simulink model "ECE545HW5_2"  (R2016a)
settings: Solver=VariableStepAuto  StartTime=0.0  StopTime=10.0  RelTol=1e-3
settings Model: Creator=clarke6  LastModifiedBy=clarke6

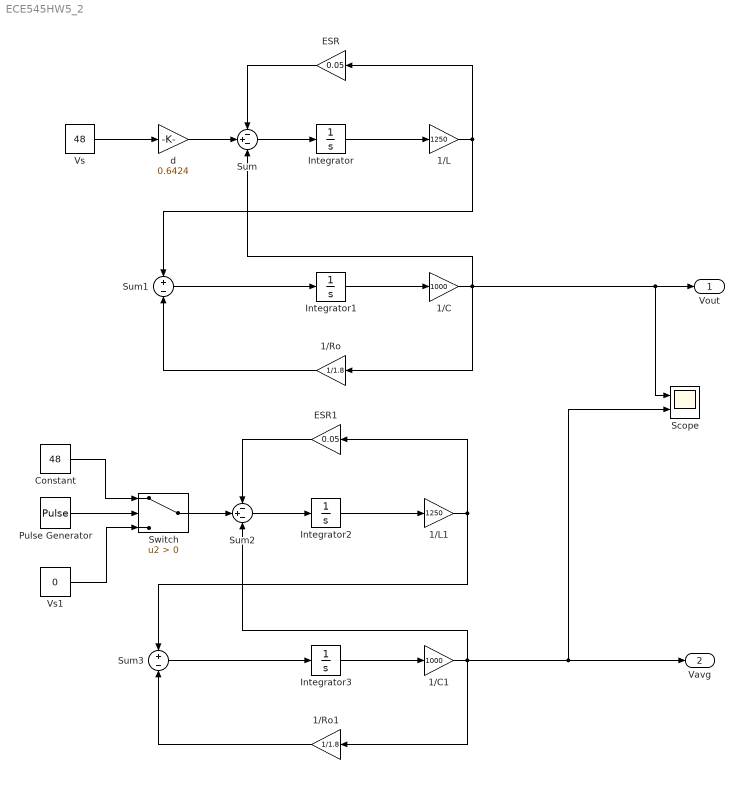
== system ECE545HW5_2 ==
  1/C : Gain  Gain=1000
  1/C1 : Gain  Gain=1000
  1/L : Gain  Gain=1250
  1/L1 : Gain  Gain=1250
  1/Ro : Gain  Gain=1/1.8
  1/Ro1 : Gain  Gain=1/1.8
  Constant : Constant  Value=48
  ESR : Gain  Gain=0.05
  ESR1 : Gain  Gain=0.05
  Integrator{,1..3} (4 alike) : Integrator
  Pulse Generator : DiscretePulseGenerator  PulseType=Time based  Period=1/20000  PulseWidth=64.24
  Scope : Scope  NumInputPorts=2
  Sum : Sum  Inputs=-+-
  Sum1 : Sum  Inputs=+|-
  Sum2 : Sum  Inputs=-+-
  Sum3 : Sum  Inputs=+|-
  Switch : Switch  Criteria=u2 > Threshold
  Vs : Constant  Value=48
  Vs1 : Constant  Value=0
  d : Gain  Gain=0.6424
  Vout : Outport
  Vavg : Outport  Port=2
  wires:
  Vs/1 -> d/1
  d/1 -> Sum/2
  Sum/1 -> Integrator/1
  Integrator/1 -> 1/L/1
  1/L/1 -> ESR/1, Sum1/1
  ESR/1 -> Sum/1
  Sum1/1 -> Integrator1/1
  Integrator1/1 -> 1/C/1
  1/C/1 -> 1/Ro/1, Vout/1, Scope/1, Sum/3
  1/Ro/1 -> Sum1/2
  Sum2/1 -> Integrator2/1
  Integrator2/1 -> 1/L1/1
  1/L1/1 -> ESR1/1, Sum3/1
  ESR1/1 -> Sum2/1
  Sum3/1 -> Integrator3/1
  Integrator3/1 -> 1/C1/1
  1/C1/1 -> Vavg/1, Scope/2, 1/Ro1/1, Sum2/3
  1/Ro1/1 -> Sum3/2
  Constant/1 -> Switch/1
  Pulse Generator/1 -> Switch/2
  Vs1/1 -> Switch/3
  Switch/1 -> Sum2/2
